simulink model "Respuesta_tiempo_delay"  (R2015a)
settings: Solver=ode45  StartTime=0.0  StopTime=200  RelTol=1e-3
values from neighbouring files (symbols this model uses):
  Kp = 35    [Comparacion_error_estacionario.m]    (also in Comparacion_error_estacionario_rampa.m; Comparacion_estabilidad.m; Comparacion_estabilidad2.m; Plot1.m)
  nn = 3    [retardo_estabilidad.m]
  r = 5    [Comparacion_error_estacionario.m]    (also in Comparacion_estabilidad.m; Comparacion_estabilidad2.m; Plot1.m; retardo_estabilidad.m)
  Ts = Tcalculado+6    (= 8)    [Comparacion_error_estacionario.m]    (also in Comparacion_error_estacionario_rampa.m; Comparacion_estabilidad.m = 30; Comparacion_estabilidad2.m = 0.5; Plot1.m = 2)
settings Model: Creator=CONTREMAR1  LastModifiedBy=CONTREMAR1

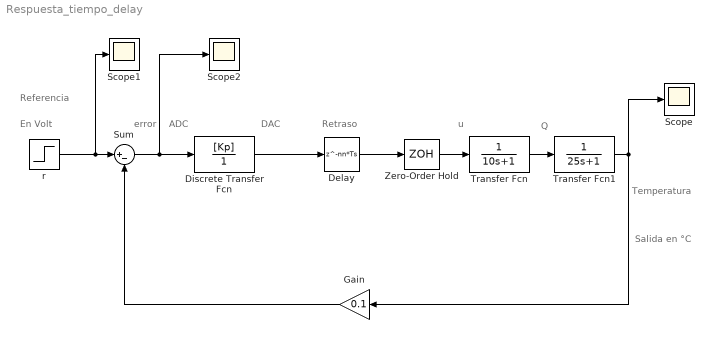
== system Respuesta_tiempo_delay ==
  note: Retraso
  note: error
  note: Salida en °C
  note: En Volt
  note: DAC
  note: ADC
  note: Temperatura
  note: Referencia
  note: u
  note: Q
  Delay : Delay  DelayLength=nn*Ts
  Discrete Transfer Fcn : DiscreteTransferFcn  Numerator=[Kp]  Denominator=[1]  SampleTime=Ts
  Gain : Gain  Gain=0.1
  Scope : Scope
      settings: SaveName=Salida
  Scope1 : Scope
      settings: SaveName=Referencia
  Scope2 : Scope
      settings: SaveName=Error
  Sum : Sum  Inputs=|+-
  Transfer Fcn : TransferFcn  Denominator=[10 1]
  Transfer Fcn1 : TransferFcn  Denominator=[25 1]
  Zero-Order Hold : ZeroOrderHold  SampleTime=Ts
  r : Step  Time=0  After=r  SampleTime=0
  wires:
  Transfer Fcn/1 -> Transfer Fcn1/1
  Zero-Order Hold/1 -> Transfer Fcn/1
  Transfer Fcn1/1 -> Gain/1, Scope/1
  r/1 -> Scope1/1, Sum/1
  Sum/1 -> Discrete Transfer Fcn/1, Scope2/1
  Gain/1 -> Sum/2
  Discrete Transfer Fcn/1 -> Delay/1
  Delay/1 -> Zero-Order Hold/1
